simulink model "mech_four_bar_trim"  (Simulink 6.0)
settings: Solver=ode45  StartTime=0.0  StopTime=10.0  RelTol=1e-3  AbsTol=1e-6
libraries: mblibv1 x11, pm_engine x1
Description:
  | MSB - Demo 2
settings Model: Creator=arnav  LastModifiedBy=batserve  ExtModeAutoUpdateStatusClock=off
settings DataIOCC: SignalLoggingName=sigsOut  Refine=5
settings OptimizationCC: BooleanDataType=off
settings DebuggingCC: CheckExecutionContextPreStartOutputMsg=on  CheckExecutionContextRuntimeOutputMsg=on  SolverPrmCheckMsg=none  UnconnectedInputMsg=none  UnconnectedOutputMsg=none  UnconnectedLineMsg=none
settings HardwareCC: TargetUnknown=on

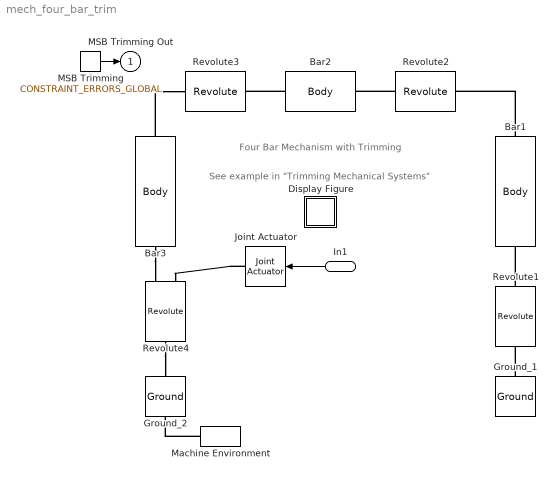
== system mech_four_bar_trim ==
  note: Four Bar Mechanism with Trimming
  note: See example in
      | "Trimming Mechanical Systems"
  In1 : Inport  Orientation=left  Port=1  LatchInput=off
  Bar1 : mblibv1/Bodies/Body  Orientation=up  PhysicalDomain=mechanical  SubClassName=Unknown  LeftPortType=workingframe  RightPortType=workingframe  LConnTagsString=CS1  RConnTagsString=CS2  DialogClass=MechanicalBodyBlock  Mass=5.357  MassUnits=kg  InertiaUnits=kg*m^2  Inertia=[1.07e-3 0 0;0 0.143 0;0 0 0.143]  Shape=Cylinder  ShapeDims=[1 1]  ShapeUnits=m  ShapeUse=false  Density=1  DensityUnits=kg/m^3  DensityUse=false  CG=Left$CG$[0.03 0.282 0]$WORLD$CS1$m$[0 0 83.1]$Euler X-Y-Z$deg$WORLD$false  WorkingFrames=Left$CS1$[0 0 0]$WORLD$ADJOINING$m$[0 0 0]$Euler X-Y-Z$deg$WORLD$true#Right$CS2$[0.063 0.597 0]$WORLD$CS1$m$[0 0 0]$Euler X-Y-Z$deg$WORLD$true
  Bar2 : mblibv1/Bodies/Body  Orientation=left  PhysicalDomain=mechanical  SubClassName=Unknown  LeftPortType=workingframe  RightPortType=workingframe  LConnTagsString=CS1  RConnTagsString=CS2  DialogClass=MechanicalBodyBlock  Mass=9.028  MassUnits=kg  InertiaUnits=kg*m^2  Inertia=[1.8e-3 0 0;0 0.678 0;0 0 0.678]  Shape=Cylinder  ShapeDims=[1 1]  ShapeUnits=m  ShapeUse=false  Density=1  DensityUnits=kg/m^3  DensityUse=false  CG=Left$CG$[-0.427 -0.242 0]$WORLD$CS1$m$[0 0 29.5]$Euler X-Y-Z$deg$WORLD$false  WorkingFrames=Left$CS1$[0 0 0]$WORLD$ADJOINING$m$[0 0 0]$Euler X-Y-Z$deg$WORLD$true#Right$CS2$[-0.87 -0.493 0]$WORLD$CS1$m$[0 0 0]$Euler X-Y-Z$deg$WORLD$true
  Bar3 : mblibv1/Bodies/Body  Orientation=down  PhysicalDomain=mechanical  SubClassName=Unknown  LeftPortType=workingframe  RightPortType=workingframe  LConnTagsString=CS1  RConnTagsString=CS2  DialogClass=MechanicalBodyBlock  Mass=0.991  MassUnits=kg  InertiaUnits=kg*m^2  Inertia=[2.06e-4 0 0;0 1.1e-3 0;0 0 1.1e-3]  Shape=Cylinder  ShapeDims=[1 1]  ShapeUnits=m  ShapeUse=false  Density=1  DensityUnits=kg/m^3  DensityUse=false  CG=Left$CG$[-0.027 -0.048 0]$WORLD$CS1$m$[0 0 60]$Euler X-Y-Z$deg$WORLD$false  WorkingFrames=Left$CS1$[0 0 0]$WORLD$ADJOINING$m$[0 0 0]$Euler X-Y-Z$deg$WORLD$true#Right$CS2$[0 0 0]$WORLD$ADJOINING$m$[0 0 0]$Euler X-Y-Z$deg$WORLD$true
  Display Figure : Subsystem  Tag=Help  Description="Help callback for trimmed four bar model: mech_four_bar_trim.  Opens Help browser to Type 19 marker at documentation for this tutorial model."
      settings: OpenFcn=pmhelpview([docroot '/toolbox/physmod/mech/mech.map'], 'mech_four_bar_trim_help');
      mask Type: Help callback
      mask Display: image(imread('info.bmp'))
  Ground_1 : mblibv1/Bodies/Ground  Orientation=up  Opaque=on  LeftPortType=env  RightPortType=workingframe  PhysicalDomain=Mechanical  DialogClass=GroundBlock  CoordPosition=[0.433 0.04 0]  CoordPositionUnits=m  StateVectorMgrId=-1  MachineId=[0 0]  ShowEnvPort=off
  Ground_2 : mblibv1/Bodies/Ground  Orientation=up  Opaque=on  LeftPortType=env  RightPortType=workingframe  PhysicalDomain=Mechanical  DialogClass=GroundBlock  CoordPosition=[-0.434 0.04 0]  CoordPositionUnits=m  StateVectorMgrId=-1  MachineId=[0 0]  ShowEnvPort=on
  Joint Actuator : mblibv1/Sensors &  Actuators/Joint Actuator  Orientation=left  Opaque=on  PhysicalDomain=Mechanical  PortType=blob  ActuationStyle=Force  AngleUnits=deg  ArcVelocityUnits=deg/s  ArcAccelerationUnits=deg/s^2  CoordPositionUnits=m  VelocityUnits=m/s  AccelerationUnits=m/s^2  ForceUnits=N  TorqueUnits=N-m  ActiveIO=off  Width=1  DialogClass=MechanicalActuatorBlock  Primitive=R1  ReferenceFrame=Absolute (INERTIAL)
  MSB Trimming : pm_engine/CONSTRAINT_ERRORS_GLOBAL
  Machine Environment : mblibv1/Bodies/Machine Environment  Tag=Factory ground  Orientation=left  DialogController=MECH.DialogSource  Opaque=on  PortType=env  PhysicalDomain=Mechanical  DialogTemplateClass=MECH.MachineEnvironment  SyncWhenCopied=off  Gravity=[0 -9.81 0]  GravityUnits=m/s^2  GravityAsSignal=off  Dimensionality=3D Only  AnalysisType=Trimming  LinearAssemblyTolerance=1e-3  LinearAssemblyToleranceUnits=m  AngularAssemblyTolerance=1e-3  AngularAssemblyToleranceUnits=rad  ConstraintSolverType=Stabilizing  ConstraintRelTolerance=1e-4  ConstraintAbsTolerance=1e-4  UseRobustSingularityHandling=off  StatePerturbationType=Adaptive  PerturbationSize=1e-3  VisualizeMachine=on
  Revolute1 : mblibv1/Joints/Revolute  Orientation=up  PhysicalDomain=mechanical  SubClassName=Unknown  LeftPortType=blob  RightPortType=blob  LConnTagsString=__newl0  RConnTagsString=__newr0  NumSAPorts=0  CutJoint=on  MarkAsCut=off  Primitives=revolute  PrimitiveProps=R1$WORLD$[0 0 1]$revolute  DialogClass=JointBlock
  Revolute2 : mblibv1/Joints/Revolute  Orientation=left  PhysicalDomain=mechanical  SubClassName=Unknown  LeftPortType=blob  RightPortType=blob  LConnTagsString=__newl0  RConnTagsString=__newr0  NumSAPorts=0  CutJoint=off  MarkAsCut=off  Primitives=revolute  PrimitiveProps=R1$WORLD$[0 0 1]$revolute  DialogClass=JointBlock
  Revolute3 : mblibv1/Joints/Revolute  Orientation=left  PhysicalDomain=mechanical  SubClassName=Unknown  LeftPortType=blob  RightPortType=blob  LConnTagsString=__newl0  RConnTagsString=__newr0  NumSAPorts=0  CutJoint=off  MarkAsCut=off  Primitives=revolute  PrimitiveProps=R1$WORLD$[0 0 1]$revolute  DialogClass=JointBlock
  Revolute4 : mblibv1/Joints/Revolute  Orientation=down  PhysicalDomain=mechanical  SubClassName=Unknown  LeftPortType=blob  RightPortType=blob  LConnTagsString=__newl0|SA1  RConnTagsString=__newr0  NumSAPorts=1  CutJoint=off  MarkAsCut=off  Primitives=revolute  PrimitiveProps=R1$WORLD$[0 0 1]$revolute  DialogClass=JointBlock
  MSB Trimming Out : Outport
  wires:
  In1/1 -> Joint Actuator/1
  MSB Trimming/1 -> MSB Trimming Out/1
  connections:
  Ground_1/RConn1 -- Revolute1/LConn1
  Revolute1/RConn1 -- Bar1/LConn1
  Bar1/RConn1 -- Revolute2/LConn1
  Revolute2/RConn1 -- Bar2/LConn1
  Bar2/RConn1 -- Revolute3/LConn1
  Bar3/LConn1 -- Revolute3/RConn1
  Bar3/RConn1 -- Revolute4/LConn1
  Revolute4/RConn1 -- Ground_2/RConn1
  Joint Actuator/RConn1 -- Revolute4/LConn2
  Machine Environment/RConn1 -- Ground_2/LConn1

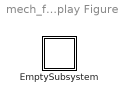
== system mech_four_bar_trim/Display Figure ==
  EmptySubsystem : Subsystem

== system mech_four_bar_trim/Display Figure/EmptySubsystem ==
